simulink model "SOGI_Test"  (R2022b)
settings: Solver=VariableStepAuto  StartTime=0.0  StopTime=1  MaxStep=1e-6  RelTol=1e-3
undefined symbols (not defined in the file): square
libraries: simulink x3
settings Model: Creator=TKWTL  LastModifiedBy=TKWTL
settings HardwareCC: ProdHWDeviceType=AMD->x86-64 (Windows64)
settings SFSimCC: SimTargetLang=C++  GPUAcceleration=on  SimDLTargetLibrary=cudnn

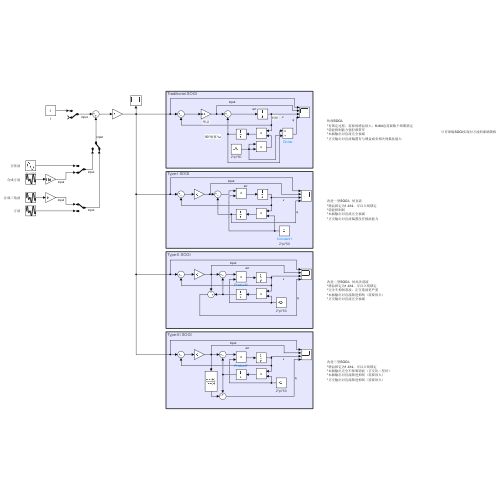
[thumbnail: Simulink's stored preview of the top-level diagram]
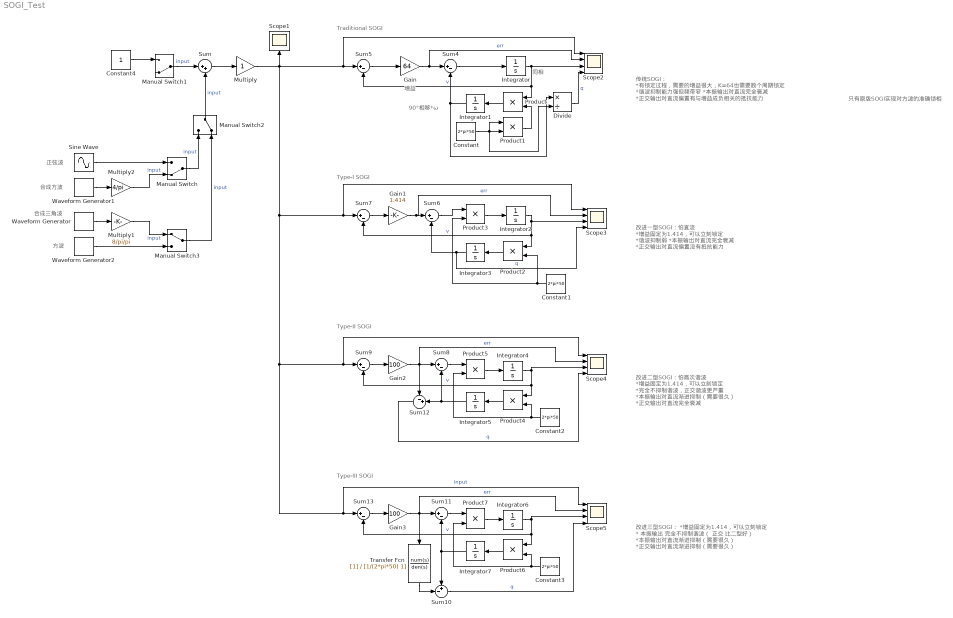
== system SOGI_Test ==
  note: 正弦波
  note: 合成方波
  note: 合成三角波
  note: 方波
  note: 只有原版SOGI实现对方波的准确锁相
  note: 改进一型SOGI：怕直流
      | *增益固定为1.414，可以立刻锁定
      | *谐波抑制弱
      | *本振输出对直流完全衰减
      | *正交输出对直流偏置没有抵抗能力
  note: 传统SOGI：
      | *有锁定过程，需要的增益很大，K=64也需要数个周期锁定
      | *谐波抑制能力强但频带窄
      | *本振输出对直流完全衰减
      | *正交输出对直流偏置有与增益成负相关的抵抗能力
  note: 增益
  note: 90°相移*ω
  note: 同相
  note: Traditional SOGI
  note: Type-I SOGI
  note: Type-II SOGI
  note: Type-III SOGI
  note: 改进二型SOGI：怕高次谐波
      | *增益固定为1.414，可以立刻锁定
      | *完全不抑制谐波，正交谐波更严重
      | *本振输出对直流渐进抑制（需要很久）
      | *正交输出对直流完全衰减
  note: 改进三型SOGI：
      | *增益固定为1.414，可以立刻锁定
      | * 本振输出 完全不抑制谐波（ 正交 比二型好）
      | *本振输出对直流渐进抑制（需要很久）
      | *正交输出对直流渐进抑制（需要很久）
  Constant{,1..3} (4 alike) : Constant  Value=2*pi*50
      settings: AttributesFormatString=%<Value>
  Constant4 : Constant
      settings: AttributesFormatString=%<Value>
  Divide : Product  Inputs=*/
  Gain : Gain  Gain=64
  Gain1 : Gain  Gain=1.414
  Gain2 : Gain  Gain=100
  Gain3 : Gain  Gain=100
  Integrator{,1..7} (8 alike) : Integrator
  Manual Switch : ManualSwitch  CurrentSetting=0
  Manual Switch1 : ManualSwitch  CurrentSetting=0
  Manual Switch2 : ManualSwitch  CurrentSetting=0
  Manual Switch3 : ManualSwitch
  Multiply : Gain
  Multiply1 : Gain  Gain=8/pi/pi
  Multiply2 : Gain  Gain=4/pi
  Product{,1..7} (8 alike) : Product
  Scope1 : Scope
  Scope{2..5} (4 alike) : Scope  NumInputPorts=4
  Sine Wave : Sin  Bias=1  Frequency=2*pi*50  SampleTime=0
      settings: AttributesFormatString=|
      | %<Frequency>
      | %<Amplitude>
      | %<Offset>
  Sum : Sum  Inputs=|++
  Sum10 : Sum  Inputs=+-|
  Sum{4..9,11,13} (8 alike) : Sum  Inputs=|+-
  Sum12 : Sum  Inputs=-+|
  Transfer Fcn : TransferFcn  Denominator=[1/(2*pi*50) 1]
  Waveform Generator : simulink/Sources/Waveform Generator  OutMin=[]  OutMax=[]  OutDataTypeStr=double  SelectedSignal=1  Signals=sin('Amplitude', 1, 'Frequency', 2*pi*50, 'Phase', 0)-sin('Amplitude', 1/9, 'Frequency', 2*pi*50*3, 'Phase', 0)+sin('Amplitude', 1/25, 'Frequency', 2*pi*50*5, 'Phase', 0)-sin('Amplitude', 1/49, 'Frequency', 2*pi*50*7, 'Phase', 0)+sin('Amplitude', 1/81, 'Frequency', 2*pi*50*9, 'Phase', 0)-sin('Amplitude', 1/121, 'Frequency', 2*pi*50*11, 'Phase', 0)  BlockNames=MultiportSwitch_300bd3e073b043c  SampleTime=1e-7
  Waveform Generator1 : simulink/Sources/Waveform Generator  OutMin=[]  OutMax=[]  OutDataTypeStr=double  SelectedSignal=1  Signals=sin('Amplitude', 1, 'Frequency', 2*pi*50, 'Phase', 0)+sin('Amplitude', 1/3, 'Frequency', 2*pi*50*3, 'Phase', 0)+sin('Amplitude', 1/5, 'Frequency', 2*pi*50*5, 'Phase', 0)+sin('Amplitude', 1/7, 'Frequency', 2*pi*50*7, 'Phase', 0)+sin('Amplitude', 1/9, 'Frequency', 2*pi*50*9, 'Phase', 0)+sin('Amplitude', 1/11, 'Frequency', 2*pi*50*11, 'Phase', 0)  BlockNames=MultiportSwitch_4d2b4e4572ef4f1  SampleTime=1e-7
  Waveform Generator2 : simulink/Sources/Waveform Generator  OutMin=[]  OutMax=[]  OutDataTypeStr=double  SelectedSignal=1  Signals=square(1,2*pi*50,0,50)  BlockNames=MultiportSwitch_62ce54ed83f1453  SampleTime=1e-7
  wires:
  Gain/1 -> Scope2/2, Sum4/1  "err"
  Sum4/1 -> Integrator/1
  Constant/1 -> Divide/2, Product1/1, Product1/2
  Product1/1 -> Product/2
  Integrator/1 -> Scope2/3, Sum5/2, Product/1  "v"
  Product/1 -> Integrator1/1
  Sum5/1 -> Gain/1
  Integrator1/1 -> Sum4/2, Divide/1
  Divide/1 -> Scope2/4  "q"
  Integrator3/1 -> Scope3/4, Sum6/2  "q"
  Product2/1 -> Integrator3/1
  Gain1/1 -> Scope3/2, Sum6/1  "err"
  Sum7/1 -> Gain1/1
  Sum12/1 -> Scope4/4  "q"
  Product4/1 -> Integrator5/1
  Integrator4/1 -> Scope4/3, Sum9/2, Product4/1  "v"
  Gain2/1 -> Sum8/1, Scope4/2, Sum12/1  "err"
  Sum9/1 -> Gain2/1
  Integrator5/1 -> Sum12/2, Sum8/2
  Constant1/1 -> Product3/2, Product2/2
  Product3/1 -> Integrator2/1
  Sum6/1 -> Product3/1
  Integrator2/1 -> Scope3/3, Sum7/2, Product2/1  "v"
  Product5/1 -> Integrator4/1
  Sum8/1 -> Product5/1
  Constant2/1 -> Product5/2, Product4/2
  Sum11/1 -> Product7/1
  Constant3/1 -> Product7/2, Product6/2
  Multiply/1 -> Scope5/1, Sum13/1, Scope4/1, Sum9/1, Scope3/1, Sum7/1, Scope1/1, Scope2/1, Sum5/1  "input"
  Gain3/1 -> Transfer Fcn/1, Sum11/1, Scope5/2  "err"
  Sum13/1 -> Gain3/1
  Product6/1 -> Integrator7/1
  Integrator6/1 -> Scope5/3, Sum13/2, Product6/1  "v"
  Integrator7/1 -> Sum10/1, Sum11/2
  Product7/1 -> Integrator6/1
  Sum10/1 -> Scope5/4  "q"
  Transfer Fcn/1 -> Sum10/2
  Sine Wave/1 -> Manual Switch/1
  Manual Switch1/1 -> Sum/1  "input"
  Constant4/1 -> Manual Switch1/1
  Sum/1 -> Multiply/1
  Manual Switch2/1 -> Sum/2  "input"
  Manual Switch3/1 -> Manual Switch2/2  "input"
  Manual Switch/1 -> Manual Switch2/1  "input"
  Waveform Generator/1 -> Multiply1/1
  Multiply1/1 -> Manual Switch3/1  "input"
  Multiply2/1 -> Manual Switch/2  "input"
  Waveform Generator1/1 -> Multiply2/1
  Waveform Generator2/1 -> Manual Switch3/2
